simulink model "Ej1"  (R2015a)
settings: Solver=ode45  StartTime=0.0  StopTime=10.0  RelTol=1e-3
libraries: cstblocks x4
settings Model: Creator=Daniel  LastModifiedBy=Daniel

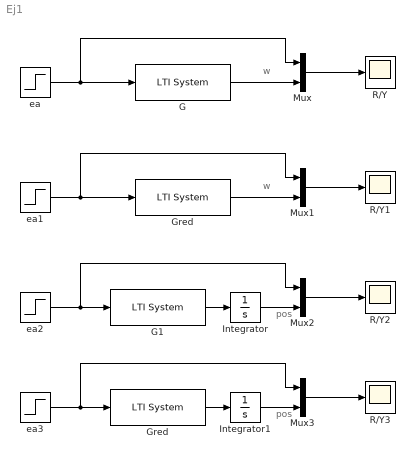
== system Ej1 ==
  note: w
  note: w
  note: pos
  note: pos
  G : cstblocks/LTI System  sys=G  IC=[]
  G1 : cstblocks/LTI System  sys=G  IC=[]
  Gred : cstblocks/LTI System  sys=Gred  IC=[]
  "Gred " : cstblocks/LTI System  sys=Gred  IC=[]
  Integrator : Integrator
  Integrator1 : Integrator
  Mux{,1..3} (4 alike) : Mux  Inputs=2
  R/Y{,1..3} (4 alike) : Scope
      R/Y settings: SaveName=w
      R/Y1 settings: SaveName=wred
      R/Y2 settings: SaveName=pos
      R/Y3 settings: SaveName=posred
  ea{,1..3} (4 alike) : Step  Time=0  SampleTime=0
  wires:
  ea/1 -> Mux/1, G/1
  G/1 -> Mux/2
  Mux/1 -> R/Y/1
  ea1/1 -> Mux1/1, "Gred "/1
  "Gred "/1 -> Mux1/2
  Mux1/1 -> R/Y1/1
  ea2/1 -> Mux2/1, G1/1
  G1/1 -> Integrator/1
  Mux2/1 -> R/Y2/1
  Integrator/1 -> Mux2/2
  ea3/1 -> Mux3/1, Gred/1
  Gred/1 -> Integrator1/1
  Mux3/1 -> R/Y3/1
  Integrator1/1 -> Mux3/2
